simulink model "RobotX_ss_acousticsSKIP_dock_odoa_ta_1021"  (R2014a)
settings: Solver=FixedStepDiscrete  StartTime=0.0  StopTime=inf  FixedStep=.25  RelTol=1e-3
undefined symbols (not defined in the file): Com1, Com2, Com3, Com4, DiscIntNeverNeededParam, standard
libraries: xpcseriallib x42, simulink x8, slrtlib x8, speedgoatlib x2, speedgoatlib_IO102 x1
(part 6 of 19)

== matlab function RobotX_ss_acousticsSKIP_dock_odoa_ta_1021/Main FSM/ODOA/SLAM1/Models for prediction/Model36/Dynamic Model ==
  data: F_surge input; F_sway input; Torque input; u input; surgeAccel output; v input; psi input; swayAccel output; yawAccel output
function [surgeAccel, swayAccel, yawAccel] = ...
    WAM_V_3DOF(F_surge, F_sway, Torque, u, v, psi)
%Written by Anderson Lebbad on August 12, 2014
%Last Edited:

%This function was heavily based off of Ariel Qu's Vel3DOF_IvanV1. It was
%rewritten for real-time use.

%This function will produce the transient output surge velocity of a
%linearized model of the USV. It is assumed that the vehicle is equivalent
%to two cylinders in the water.

%%%%%DEFINED VARIABLE%%%%%%
%
%   Xext = Thrust from motors
%   Next = Moment from motor
%   m = Mass of vehicle
%   Xudot = Added mass in surge direction
%   Yvdot = Added mass in sway direction
%   Nrdot = Added mass from yaw
%   xg = offset from center of gravity
%   rho = density of seawater
%   S = wetted surface area
%   R = Reynolds number
%   Cd = Coefficient of drag
%   Cdc = Coefficient of drag for sway
%   nu = Kinematic viscosity
%   L = Length overall
%   T = draft
%   B = beam
%   SA = Surface area of cylinder experiencing sway
%   Iz = moment of inertia about Z axis
%
%%%%%%

% Force/Mometns from thrusters & control surfaces...

tau = [F_surge; F_sway; Torque];

% Calculate yaw rate
persistent lastHeading
if isempty(lastHeading)
    lastHeading = psi;
end
%Sample time
ts = .1;

r = (psi - lastHeading)/ts;

% Velocity & Angular velocity vectors
vel = [u; v; 0];
omega = [0; 0; r];

%define variables
m = 145.7;         % Total mass [kg] - reduced from 102
rho = 1025.9;   % density of seawater [kg/m^3]
L = 3.91*0.85;  % Length on the waterline [m]
B = 0.426;       % Demihull beam [m]
T = B*0.2;        % Draft of the demihull [m]
p_bar = 1.0; % sidehull separation - from centerplane vessel to centerplane demihull
Iz = 262.181;    % Mass moment of inertia about z-axis [kg*m^2]
xg = 0;         % Body-Fixed coordinate system taken to be center of gravity
yg = 0;         % Symmetrical Vessel
Cd = 1.1;       % Drag coefficient for a lateral cylinder
LCG = 1.485;        % Need to know where LCG wrt stern

% Vector location of port and starboard hulls
r_port = [-LCG; -p_bar; 0];   
r_stbd = [-LCG; p_bar; 0];

% Port and starboard hull velocities
vel_port = vel + cross(omega,r_port);
vel_stbd = vel + cross(omega,r_stbd);

u_port = vel_port(1);
u_stbd = vel_stbd(1);

% Port and starboard state vectors
state_port = vel_port + omega;
state_stbd = vel_stbd + omega;

%% Added Mass
% Estimated for each hull, then multiplied by 2 to account for both hulls
Xudot = -0.05*m;

%Using strip theory to estimate added mass coefficients
Nrdot = -(4.75/2*pi*rho*p_bar*T^4 + pi*rho*T^2*((L - LCG)^3 + LCG^3)/3);
Nvdot = - pi*rho*T^2*((L - LCG)^2 - LCG^2)/2;

Yrdot = Nvdot;
Yvdot = -rho*pi*T^2*L;

% Multiply by 2:
Xudot = 2*Xudot;
Nrdot = 2*Nrdot;
Nvdot = 2*Nvdot;
Yrdot = 2*Yrdot;
Yvdot = 2*Yvdot;

%Calculate Coefficient of Drag for Sway from 1950 SNAME approximation
Cdc= 1.1 + 0.0045*L/T - 0.1*B/T + 0.016*(B/T)^2;
SA = 2*pi/4*T*L; %projected area of pontoon for two pontoons

%% Linear Drag Terms
%Total Speed
U = sqrt(u^2+v^2);

Xu = 0;
Yv = -0.5*rho*abs(v)*2*Cdc*SA; %20 was the last working number %from SNAME 1950, x2 for two cylinders
%Nr = -0.5*pi*rho*U*T^2*L^2;
Nr = -pi*rho*U*T^2*L^2*.065;
Nv = -pi*rho*U*T^2*L*.01;
Yr = pi*rho*U*T^2*L*0.2;  %from Newman approximation in Lewandowski

%% Nonlinear Drag Terms

% Drag and Moment due to drag on entire vessel - includes nonlinear and
% linear drag terms
D_port = 0.5*(0.44*u_port^3 - 0.01*u_port^2 + 19*u_port);     % Can assume that this equation also takes into account Xu - so set Xu=0
D_stbd = 0.5*(0.44*u_stbd^3 - 0.01*u_stbd^2 + 19*u_stbd);     % Can assume that this equation also takes into account Xu - so set Xu=0

tau_drag = [-(D_port + D_stbd); 0; (D_stbd - D_port)*p_bar];

Xuu = 0;

%% Maneuvering Coefficient Matrices
% Added Mass Matrix
M = [(m - Xudot)      0              0;...
    0               (m - Yvdot)     (m*xg - Yrdot);...
    0               (m*xg - Nvdot)  (Iz - Nrdot)];

%Centripetal and Added Mass Centripetal force matrices
% C_RB = [
%     0                  0                0
%     0                  0                0
%     0                  0                0
%     ];

% C_RB = [
%     0                  0                -m*(xg*r + v)
%     0                  0                -m*(yg*r - u)
%     m*(xg*r + v)       m*(yg*r - u)     0
%     ];

% C_A = -[ %negative originally
%     0                               0           0
%     0                               0           0
%     0                               0           0
%     ];

% Negating centripetal acceleration for test
C_RB = 0;
C_A = 0;

D = -[Xu  0   0;...
      0   Yv  Yr;...
      0   Nv  Nr];

% Nonlinear Drag Coefficients
D_N = -[Xuu*u   0                       0;...
        0       0                       0;...
        0       0                       0];
    
%% Calculate the port and starboard force vectors
tau_port = -(C_RB + C_A + D + D_N)*state_port;
tau_stbd = -(C_RB + C_A + D + D_N)*state_stbd;


%% Sum the force vectors
tau_tot = tau + tau_drag + tau_port + tau_stbd...
    + cross(r_port,[tau_port(1);tau_port(2);0]) + ...
    cross(r_stbd,[tau_stbd(1);tau_stbd(2);0]);

% Calculate the time derivative of the state vector

accel = M\tau_tot;

%% Separate output

surgeAccel = accel(1);
swayAccel = accel(2);
yawAccel = accel(3);

end

== matlab function RobotX_ss_acousticsSKIP_dock_odoa_ta_1021/Main FSM/ODOA/SLAM1/Models for prediction/Model39/Stbd Thruster Model ==
  data: stbdMP input; F_surge output; stbdAzimuth input; F_sway output; Torque output
function [F_surge,F_sway,Torque]  = StarBoardThruster(stbdMP,stbdAzimuth)
%Approximation for Starboard Force and Moment with the input motor power
%and azimuth angle of thruster

%Longitudinal distance from center of mass
longDist =1.007;           %m

%Axial distance from center of mass
axialDist=1.485;            %m

%% Piece-wise thrust calculation

if stbdMP <= -51.0119
    F = .9140*stbdMP + 40;
elseif stbdMP >= 26.8367
    F = 1.658*stbdMP - 41.01;
else
    F = .12987*stbdMP;
end

%% Force components
F_surge=F*cos(stbdAzimuth*pi/180);       %N
F_sway=F*sin(stbdAzimuth*pi/180);       %N

%% Torque calculation

Torque = -F_surge*longDist - F_sway*axialDist;   %N.m

end

== matlab function RobotX_ss_acousticsSKIP_dock_odoa_ta_1021/Main FSM/ODOA/SLAM1/Models for prediction/Model4/Dynamic Model ==
  data: F_surge input; F_sway input; Torque input; u input; surgeAccel output; v input; psi input; swayAccel output; yawAccel output
function [surgeAccel, swayAccel, yawAccel] = ...
    WAM_V_3DOF(F_surge, F_sway, Torque, u, v, psi)
%Written by Anderson Lebbad on August 12, 2014
%Last Edited:

%This function was heavily based off of Ariel Qu's Vel3DOF_IvanV1. It was
%rewritten for real-time use.

%This function will produce the transient output surge velocity of a
%linearized model of the USV. It is assumed that the vehicle is equivalent
%to two cylinders in the water.

%%%%%DEFINED VARIABLE%%%%%%
%
%   Xext = Thrust from motors
%   Next = Moment from motor
%   m = Mass of vehicle
%   Xudot = Added mass in surge direction
%   Yvdot = Added mass in sway direction
%   Nrdot = Added mass from yaw
%   xg = offset from center of gravity
%   rho = density of seawater
%   S = wetted surface area
%   R = Reynolds number
%   Cd = Coefficient of drag
%   Cdc = Coefficient of drag for sway
%   nu = Kinematic viscosity
%   L = Length overall
%   T = draft
%   B = beam
%   SA = Surface area of cylinder experiencing sway
%   Iz = moment of inertia about Z axis
%
%%%%%%

% Force/Mometns from thrusters & control surfaces...

tau = [F_surge; F_sway; Torque];

% Calculate yaw rate
persistent lastHeading
if isempty(lastHeading)
    lastHeading = psi;
end
%Sample time
ts = .1;

r = (psi - lastHeading)/ts;

% Velocity & Angular velocity vectors
vel = [u; v; 0];
omega = [0; 0; r];

%define variables
m = 145.7;         % Total mass [kg] - reduced from 102
rho = 1025.9;   % density of seawater [kg/m^3]
L = 3.91*0.85;  % Length on the waterline [m]
B = 0.426;       % Demihull beam [m]
T = B*0.2;        % Draft of the demihull [m]
p_bar = 1.0; % sidehull separation - from centerplane vessel to centerplane demihull
Iz = 262.181;    % Mass moment of inertia about z-axis [kg*m^2]
xg = 0;         % Body-Fixed coordinate system taken to be center of gravity
yg = 0;         % Symmetrical Vessel
Cd = 1.1;       % Drag coefficient for a lateral cylinder
LCG = 1.485;        % Need to know where LCG wrt stern

% Vector location of port and starboard hulls
r_port = [-LCG; -p_bar; 0];   
r_stbd = [-LCG; p_bar; 0];

% Port and starboard hull velocities
vel_port = vel + cross(omega,r_port);
vel_stbd = vel + cross(omega,r_stbd);

u_port = vel_port(1);
u_stbd = vel_stbd(1);

% Port and starboard state vectors
state_port = vel_port + omega;
state_stbd = vel_stbd + omega;

%% Added Mass
% Estimated for each hull, then multiplied by 2 to account for both hulls
Xudot = -0.05*m;

%Using strip theory to estimate added mass coefficients
Nrdot = -(4.75/2*pi*rho*p_bar*T^4 + pi*rho*T^2*((L - LCG)^3 + LCG^3)/3);
Nvdot = - pi*rho*T^2*((L - LCG)^2 - LCG^2)/2;

Yrdot = Nvdot;
Yvdot = -rho*pi*T^2*L;

% Multiply by 2:
Xudot = 2*Xudot;
Nrdot = 2*Nrdot;
Nvdot = 2*Nvdot;
Yrdot = 2*Yrdot;
Yvdot = 2*Yvdot;

%Calculate Coefficient of Drag for Sway from 1950 SNAME approximation
Cdc= 1.1 + 0.0045*L/T - 0.1*B/T + 0.016*(B/T)^2;
SA = 2*pi/4*T*L; %projected area of pontoon for two pontoons

%% Linear Drag Terms
%Total Speed
U = sqrt(u^2+v^2);

Xu = 0;
Yv = -0.5*rho*abs(v)*2*Cdc*SA; %20 was the last working number %from SNAME 1950, x2 for two cylinders
%Nr = -0.5*pi*rho*U*T^2*L^2;
Nr = -pi*rho*U*T^2*L^2*.065;
Nv = -pi*rho*U*T^2*L*.01;
Yr = pi*rho*U*T^2*L*0.2;  %from Newman approximation in Lewandowski

%% Nonlinear Drag Terms

% Drag and Moment due to drag on entire vessel - includes nonlinear and
% linear drag terms
D_port = 0.5*(0.44*u_port^3 - 0.01*u_port^2 + 19*u_port);     % Can assume that this equation also takes into account Xu - so set Xu=0
D_stbd = 0.5*(0.44*u_stbd^3 - 0.01*u_stbd^2 + 19*u_stbd);     % Can assume that this equation also takes into account Xu - so set Xu=0

tau_drag = [-(D_port + D_stbd); 0; (D_stbd - D_port)*p_bar];

Xuu = 0;

%% Maneuvering Coefficient Matrices
% Added Mass Matrix
M = [(m - Xudot)      0              0;...
    0               (m - Yvdot)     (m*xg - Yrdot);...
    0               (m*xg - Nvdot)  (Iz - Nrdot)];

%Centripetal and Added Mass Centripetal force matrices
% C_RB = [
%     0                  0                0
%     0                  0                0
%     0                  0                0
%     ];

% C_RB = [
%     0                  0                -m*(xg*r + v)
%     0                  0                -m*(yg*r - u)
%     m*(xg*r + v)       m*(yg*r - u)     0
%     ];

% C_A = -[ %negative originally
%     0                               0           0
%     0                               0           0
%     0                               0           0
%     ];

% Negating centripetal acceleration for test
C_RB = 0;
C_A = 0;

D = -[Xu  0   0;...
      0   Yv  Yr;...
      0   Nv  Nr];

% Nonlinear Drag Coefficients
D_N = -[Xuu*u   0                       0;...
        0       0                       0;...
        0       0                       0];
    
%% Calculate the port and starboard force vectors
tau_port = -(C_RB + C_A + D + D_N)*state_port;
tau_stbd = -(C_RB + C_A + D + D_N)*state_stbd;


%% Sum the force vectors
tau_tot = tau + tau_drag + tau_port + tau_stbd...
    + cross(r_port,[tau_port(1);tau_port(2);0]) + ...
    cross(r_stbd,[tau_stbd(1);tau_stbd(2);0]);

% Calculate the time derivative of the state vector

accel = M\tau_tot;

%% Separate output

surgeAccel = accel(1);
swayAccel = accel(2);
yawAccel = accel(3);

end

== matlab function RobotX_ss_acousticsSKIP_dock_odoa_ta_1021/Main FSM/ODOA/SLAM1/Models for prediction/Model42/Stbd Thruster Model ==
  data: stbdMP input; F_surge output; stbdAzimuth input; F_sway output; Torque output
function [F_surge,F_sway,Torque]  = StarBoardThruster(stbdMP,stbdAzimuth)
%Approximation for Starboard Force and Moment with the input motor power
%and azimuth angle of thruster

%Longitudinal distance from center of mass
longDist =1.007;           %m

%Axial distance from center of mass
axialDist=1.485;            %m

%% Piece-wise thrust calculation

if stbdMP <= -51.0119
    F = .9140*stbdMP + 40;
elseif stbdMP >= 26.8367
    F = 1.658*stbdMP - 41.01;
else
    F = .12987*stbdMP;
end

%% Force components
F_surge=F*cos(stbdAzimuth*pi/180);       %N
F_sway=F*sin(stbdAzimuth*pi/180);       %N

%% Torque calculation

Torque = -F_surge*longDist - F_sway*axialDist;   %N.m

end

== matlab function RobotX_ss_acousticsSKIP_dock_odoa_ta_1021/Main FSM/ODOA/SLAM1/Models for prediction/Model43/Non-Holonomic Constraint ==
  data: time input; surgeAccel input; NEyaw output; swayAccel input; YawAccel input; u input; v input; gyrz input; psi input; X input; Y input
function NEyaw  = nonHolonomicNE(time,surgeAccel,swayAccel,YawAccel,u,v,gyrz,psi,X,Y)
%Written by Anderson Lebbad on August 12, 2014
%Last Edited:

%This function estimates the velocities for a new pose based off the 
%velocities and heading calculated from the dynamic model, and the current 
%pose. Uses a non-holonomic constraint for estimation.

%% Find time elapsed for integration

ts = .1;
persistent uPrev vPrev gyrzPrev psiPrev xPrev yPrev

%Initialize
if isempty(uPrev)
    uPrev = [u time];
    vPrev = [v time];
    gyrzPrev = [gyrz time];
    psiPrev = [psi time];
    xPrev = [X time];
    yPrev = [Y time];
end
    
%Update if change
if uPrev(1) ~= u
    uPrev = [u time];
end
if vPrev(1) ~= v
    vPrev = [v time];
end
if gyrzPrev(1) ~= gyrz
    gyrzPrev = [gyrz time];
end
if psiPrev(1) ~= psi
    psiPrev = [psi time];
end
if xPrev(1) ~= X
    xPrev = [X time];
end
if yPrev(1) ~= Y
    yPrev = [Y time];
end

%evaluate elapsed
uTime = ts + time - uPrev(2);
vTime = ts + time - vPrev(2);
gyrzTime = ts + time - gyrzPrev(2);
psiTime = ts + time - psiPrev(2);
xTime = ts + time - xPrev(2);
yTime = ts + time - yPrev(2);

%% Integrate inputs
surgeVel = u + surgeAccel*uTime/2;
swayVel = v + swayAccel*vTime/2;
yawVel = gyrz + YawAccel*gyrzTime/2;
yaw = psi + yawVel*psiTime/2;


%% Apply Non-holonomic constraint for NE velocities
Xd = surgeVel*cos(yaw*pi/180) - swayVel*sin(yaw*pi/180);
Yd = surgeVel*sin(yaw*pi/180) + swayVel*cos(yaw*pi/180);

%% Integrate to output NE coordinates
N = X + Xd*xTime/2;
E = Y + Yd*yTime/2;

NEyaw = [N;E;yaw];

end

== matlab function RobotX_ss_acousticsSKIP_dock_odoa_ta_1021/Main FSM/ODOA/SLAM1/Models for prediction/Model44/Port Thruster Model ==
  data: portMP input; F_surge output; portAzimuth input; F_sway output; Torque output
function [F_surge,F_sway,Torque]  = PortThruster(portMP,portAzimuth)
%Approximation for Starboard Force and Moment with the input motor power
%and azimuth angle of thruster

%Longitudinal distance from center of mass
longDist =1.007;           %m

%Axial distance from center of mass
axialDist=1.485;            %m

%% Piece-wise thrust calculation

if portMP <= -51.0119
    F = .9140*portMP + 40;
elseif portMP >= 26.8367
    F = 1.658*portMP - 41.01;
else
    F = .12987*portMP;
end

%% Force components
F_surge=F*cos(portAzimuth*pi/180);       %N
F_sway=F*sin(portAzimuth*pi/180);       %N

%% Torque calculation

Torque = F_surge*longDist - F_sway*axialDist;   %N.m

end

== matlab function RobotX_ss_acousticsSKIP_dock_odoa_ta_1021/Main FSM/ODOA/SLAM1/Models for prediction/Model44/move_part ==
  data: PtThrust input; portMP output; PtAzimuth input; StThrust input; StAzimuth input; noiseLevel input; portAzimuth output; stbdMP output; stbdAzimuth output
function [portMP,portAzimuth,stbdMP,stbdAzimuth] = addNoise(PtThrust,...
    PtAzimuth,StThrust,StAzimuth,noiseLevel)
%Written By Anderson Lebbad on September 16, 2014
%Last Edited By:

%This function adds gaussian noise to the inputs for a particular particles
%model

portMP = normrnd(PtThrust, noiseLevel);
portAzimuth = normrnd(PtAzimuth, noiseLevel);
stbdMP = normrnd(StThrust, noiseLevel);
stbdAzimuth = normrnd(StAzimuth, noiseLevel);

end

== matlab function RobotX_ss_acousticsSKIP_dock_odoa_ta_1021/Main FSM/ODOA/SLAM1/Models for prediction/Model45/Dynamic Model ==
  data: F_surge input; F_sway input; Torque input; u input; surgeAccel output; v input; psi input; swayAccel output; yawAccel output
function [surgeAccel, swayAccel, yawAccel] = ...
    WAM_V_3DOF(F_surge, F_sway, Torque, u, v, psi)
%Written by Anderson Lebbad on August 12, 2014
%Last Edited:

%This function was heavily based off of Ariel Qu's Vel3DOF_IvanV1. It was
%rewritten for real-time use.

%This function will produce the transient output surge velocity of a
%linearized model of the USV. It is assumed that the vehicle is equivalent
%to two cylinders in the water.

%%%%%DEFINED VARIABLE%%%%%%
%
%   Xext = Thrust from motors
%   Next = Moment from motor
%   m = Mass of vehicle
%   Xudot = Added mass in surge direction
%   Yvdot = Added mass in sway direction
%   Nrdot = Added mass from yaw
%   xg = offset from center of gravity
%   rho = density of seawater
%   S = wetted surface area
%   R = Reynolds number
%   Cd = Coefficient of drag
%   Cdc = Coefficient of drag for sway
%   nu = Kinematic viscosity
%   L = Length overall
%   T = draft
%   B = beam
%   SA = Surface area of cylinder experiencing sway
%   Iz = moment of inertia about Z axis
%
%%%%%%

% Force/Mometns from thrusters & control surfaces...

tau = [F_surge; F_sway; Torque];

% Calculate yaw rate
persistent lastHeading
if isempty(lastHeading)
    lastHeading = psi;
end
%Sample time
ts = .1;

r = (psi - lastHeading)/ts;

% Velocity & Angular velocity vectors
vel = [u; v; 0];
omega = [0; 0; r];

%define variables
m = 145.7;         % Total mass [kg] - reduced from 102
rho = 1025.9;   % density of seawater [kg/m^3]
L = 3.91*0.85;  % Length on the waterline [m]
B = 0.426;       % Demihull beam [m]
T = B*0.2;        % Draft of the demihull [m]
p_bar = 1.0; % sidehull separation - from centerplane vessel to centerplane demihull
Iz = 262.181;    % Mass moment of inertia about z-axis [kg*m^2]
xg = 0;         % Body-Fixed coordinate system taken to be center of gravity
yg = 0;         % Symmetrical Vessel
Cd = 1.1;       % Drag coefficient for a lateral cylinder
LCG = 1.485;        % Need to know where LCG wrt stern

% Vector location of port and starboard hulls
r_port = [-LCG; -p_bar; 0];   
r_stbd = [-LCG; p_bar; 0];

% Port and starboard hull velocities
vel_port = vel + cross(omega,r_port);
vel_stbd = vel + cross(omega,r_stbd);

u_port = vel_port(1);
u_stbd = vel_stbd(1);

% Port and starboard state vectors
state_port = vel_port + omega;
state_stbd = vel_stbd + omega;

%% Added Mass
% Estimated for each hull, then multiplied by 2 to account for both hulls
Xudot = -0.05*m;

%Using strip theory to estimate added mass coefficients
Nrdot = -(4.75/2*pi*rho*p_bar*T^4 + pi*rho*T^2*((L - LCG)^3 + LCG^3)/3);
Nvdot = - pi*rho*T^2*((L - LCG)^2 - LCG^2)/2;

Yrdot = Nvdot;
Yvdot = -rho*pi*T^2*L;

% Multiply by 2:
Xudot = 2*Xudot;
Nrdot = 2*Nrdot;
Nvdot = 2*Nvdot;
Yrdot = 2*Yrdot;
Yvdot = 2*Yvdot;

%Calculate Coefficient of Drag for Sway from 1950 SNAME approximation
Cdc= 1.1 + 0.0045*L/T - 0.1*B/T + 0.016*(B/T)^2;
SA = 2*pi/4*T*L; %projected area of pontoon for two pontoons

%% Linear Drag Terms
%Total Speed
U = sqrt(u^2+v^2);

Xu = 0;
Yv = -0.5*rho*abs(v)*2*Cdc*SA; %20 was the last working number %from SNAME 1950, x2 for two cylinders
%Nr = -0.5*pi*rho*U*T^2*L^2;
Nr = -pi*rho*U*T^2*L^2*.065;
Nv = -pi*rho*U*T^2*L*.01;
Yr = pi*rho*U*T^2*L*0.2;  %from Newman approximation in Lewandowski

%% Nonlinear Drag Terms

% Drag and Moment due to drag on entire vessel - includes nonlinear and
% linear drag terms
D_port = 0.5*(0.44*u_port^3 - 0.01*u_port^2 + 19*u_port);     % Can assume that this equation also takes into account Xu - so set Xu=0
D_stbd = 0.5*(0.44*u_stbd^3 - 0.01*u_stbd^2 + 19*u_stbd);     % Can assume that this equation also takes into account Xu - so set Xu=0

tau_drag = [-(D_port + D_stbd); 0; (D_stbd - D_port)*p_bar];

Xuu = 0;

%% Maneuvering Coefficient Matrices
% Added Mass Matrix
M = [(m - Xudot)      0              0;...
    0               (m - Yvdot)     (m*xg - Yrdot);...
    0               (m*xg - Nvdot)  (Iz - Nrdot)];

%Centripetal and Added Mass Centripetal force matrices
% C_RB = [
%     0                  0                0
%     0                  0                0
%     0                  0                0
%     ];

% C_RB = [
%     0                  0                -m*(xg*r + v)
%     0                  0                -m*(yg*r - u)
%     m*(xg*r + v)       m*(yg*r - u)     0
%     ];

% C_A = -[ %negative originally
%     0                               0           0
%     0                               0           0
%     0                               0           0
%     ];

% Negating centripetal acceleration for test
C_RB = 0;
C_A = 0;

D = -[Xu  0   0;...
      0   Yv  Yr;...
      0   Nv  Nr];

% Nonlinear Drag Coefficients
D_N = -[Xuu*u   0                       0;...
        0       0                       0;...
        0       0                       0];
    
%% Calculate the port and starboard force vectors
tau_port = -(C_RB + C_A + D + D_N)*state_port;
tau_stbd = -(C_RB + C_A + D + D_N)*state_stbd;


%% Sum the force vectors
tau_tot = tau + tau_drag + tau_port + tau_stbd...
    + cross(r_port,[tau_port(1);tau_port(2);0]) + ...
    cross(r_stbd,[tau_stbd(1);tau_stbd(2);0]);

% Calculate the time derivative of the state vector

accel = M\tau_tot;

%% Separate output

surgeAccel = accel(1);
swayAccel = accel(2);
yawAccel = accel(3);

end

== matlab function RobotX_ss_acousticsSKIP_dock_odoa_ta_1021/Main FSM/ODOA/SLAM1/Models for prediction/Model48/Stbd Thruster Model ==
  data: stbdMP input; F_surge output; stbdAzimuth input; F_sway output; Torque output
function [F_surge,F_sway,Torque]  = StarBoardThruster(stbdMP,stbdAzimuth)
%Approximation for Starboard Force and Moment with the input motor power
%and azimuth angle of thruster

%Longitudinal distance from center of mass
longDist =1.007;           %m

%Axial distance from center of mass
axialDist=1.485;            %m

%% Piece-wise thrust calculation

if stbdMP <= -51.0119
    F = .9140*stbdMP + 40;
elseif stbdMP >= 26.8367
    F = 1.658*stbdMP - 41.01;
else
    F = .12987*stbdMP;
end

%% Force components
F_surge=F*cos(stbdAzimuth*pi/180);       %N
F_sway=F*sin(stbdAzimuth*pi/180);       %N

%% Torque calculation

Torque = -F_surge*longDist - F_sway*axialDist;   %N.m

end

== matlab function RobotX_ss_acousticsSKIP_dock_odoa_ta_1021/Main FSM/ODOA/SLAM1/Models for prediction/Model49/Dynamic Model ==
  data: F_surge input; F_sway input; Torque input; u input; surgeAccel output; v input; psi input; swayAccel output; yawAccel output
function [surgeAccel, swayAccel, yawAccel] = ...
    WAM_V_3DOF(F_surge, F_sway, Torque, u, v, psi)
%Written by Anderson Lebbad on August 12, 2014
%Last Edited:

%This function was heavily based off of Ariel Qu's Vel3DOF_IvanV1. It was
%rewritten for real-time use.

%This function will produce the transient output surge velocity of a
%linearized model of the USV. It is assumed that the vehicle is equivalent
%to two cylinders in the water.

%%%%%DEFINED VARIABLE%%%%%%
%
%   Xext = Thrust from motors
%   Next = Moment from motor
%   m = Mass of vehicle
%   Xudot = Added mass in surge direction
%   Yvdot = Added mass in sway direction
%   Nrdot = Added mass from yaw
%   xg = offset from center of gravity
%   rho = density of seawater
%   S = wetted surface area
%   R = Reynolds number
%   Cd = Coefficient of drag
%   Cdc = Coefficient of drag for sway
%   nu = Kinematic viscosity
%   L = Length overall
%   T = draft
%   B = beam
%   SA = Surface area of cylinder experiencing sway
%   Iz = moment of inertia about Z axis
%
%%%%%%

% Force/Mometns from thrusters & control surfaces...

tau = [F_surge; F_sway; Torque];

% Calculate yaw rate
persistent lastHeading
if isempty(lastHeading)
    lastHeading = psi;
end
%Sample time
ts = .1;

r = (psi - lastHeading)/ts;

% Velocity & Angular velocity vectors
vel = [u; v; 0];
omega = [0; 0; r];

%define variables
m = 145.7;         % Total mass [kg] - reduced from 102
rho = 1025.9;   % density of seawater [kg/m^3]
L = 3.91*0.85;  % Length on the waterline [m]
B = 0.426;       % Demihull beam [m]
T = B*0.2;        % Draft of the demihull [m]
p_bar = 1.0; % sidehull separation - from centerplane vessel to centerplane demihull
Iz = 262.181;    % Mass moment of inertia about z-axis [kg*m^2]
xg = 0;         % Body-Fixed coordinate system taken to be center of gravity
yg = 0;         % Symmetrical Vessel
Cd = 1.1;       % Drag coefficient for a lateral cylinder
LCG = 1.485;        % Need to know where LCG wrt stern

% Vector location of port and starboard hulls
r_port = [-LCG; -p_bar; 0];   
r_stbd = [-LCG; p_bar; 0];

% Port and starboard hull velocities
vel_port = vel + cross(omega,r_port);
vel_stbd = vel + cross(omega,r_stbd);

u_port = vel_port(1);
u_stbd = vel_stbd(1);

% Port and starboard state vectors
state_port = vel_port + omega;
state_stbd = vel_stbd + omega;

%% Added Mass
% Estimated for each hull, then multiplied by 2 to account for both hulls
Xudot = -0.05*m;

%Using strip theory to estimate added mass coefficients
Nrdot = -(4.75/2*pi*rho*p_bar*T^4 + pi*rho*T^2*((L - LCG)^3 + LCG^3)/3);
Nvdot = - pi*rho*T^2*((L - LCG)^2 - LCG^2)/2;

Yrdot = Nvdot;
Yvdot = -rho*pi*T^2*L;

% Multiply by 2:
Xudot = 2*Xudot;
Nrdot = 2*Nrdot;
Nvdot = 2*Nvdot;
Yrdot = 2*Yrdot;
Yvdot = 2*Yvdot;

%Calculate Coefficient of Drag for Sway from 1950 SNAME approximation
Cdc= 1.1 + 0.0045*L/T - 0.1*B/T + 0.016*(B/T)^2;
SA = 2*pi/4*T*L; %projected area of pontoon for two pontoons

%% Linear Drag Terms
%Total Speed
U = sqrt(u^2+v^2);

Xu = 0;
Yv = -0.5*rho*abs(v)*2*Cdc*SA; %20 was the last working number %from SNAME 1950, x2 for two cylinders
%Nr = -0.5*pi*rho*U*T^2*L^2;
Nr = -pi*rho*U*T^2*L^2*.065;
Nv = -pi*rho*U*T^2*L*.01;
Yr = pi*rho*U*T^2*L*0.2;  %from Newman approximation in Lewandowski

%% Nonlinear Drag Terms

% Drag and Moment due to drag on entire vessel - includes nonlinear and
% linear drag terms
D_port = 0.5*(0.44*u_port^3 - 0.01*u_port^2 + 19*u_port);     % Can assume that this equation also takes into account Xu - so set Xu=0
D_stbd = 0.5*(0.44*u_stbd^3 - 0.01*u_stbd^2 + 19*u_stbd);     % Can assume that this equation also takes into account Xu - so set Xu=0

tau_drag = [-(D_port + D_stbd); 0; (D_stbd - D_port)*p_bar];

Xuu = 0;

%% Maneuvering Coefficient Matrices
% Added Mass Matrix
M = [(m - Xudot)      0              0;...
    0               (m - Yvdot)     (m*xg - Yrdot);...
    0               (m*xg - Nvdot)  (Iz - Nrdot)];

%Centripetal and Added Mass Centripetal force matrices
% C_RB = [
%     0                  0                0
%     0                  0                0
%     0                  0                0
%     ];

% C_RB = [
%     0                  0                -m*(xg*r + v)
%     0                  0                -m*(yg*r - u)
%     m*(xg*r + v)       m*(yg*r - u)     0
%     ];

% C_A = -[ %negative originally
%     0                               0           0
%     0                               0           0
%     0                               0           0
%     ];

% Negating centripetal acceleration for test
C_RB = 0;
C_A = 0;

D = -[Xu  0   0;...
      0   Yv  Yr;...
      0   Nv  Nr];

% Nonlinear Drag Coefficients
D_N = -[Xuu*u   0                       0;...
        0       0                       0;...
        0       0                       0];
    
%% Calculate the port and starboard force vectors
tau_port = -(C_RB + C_A + D + D_N)*state_port;
tau_stbd = -(C_RB + C_A + D + D_N)*state_stbd;


%% Sum the force vectors
tau_tot = tau + tau_drag + tau_port + tau_stbd...
    + cross(r_port,[tau_port(1);tau_port(2);0]) + ...
    cross(r_stbd,[tau_stbd(1);tau_stbd(2);0]);

% Calculate the time derivative of the state vector

accel = M\tau_tot;

%% Separate output

surgeAccel = accel(1);
swayAccel = accel(2);
yawAccel = accel(3);

end

== matlab function RobotX_ss_acousticsSKIP_dock_odoa_ta_1021/Main FSM/ODOA/SLAM1/Models for prediction/Model6/Stbd Thruster Model ==
  data: stbdMP input; F_surge output; stbdAzimuth input; F_sway output; Torque output
function [F_surge,F_sway,Torque]  = StarBoardThruster(stbdMP,stbdAzimuth)
%Approximation for Starboard Force and Moment with the input motor power
%and azimuth angle of thruster

%Longitudinal distance from center of mass
longDist =1.007;           %m

%Axial distance from center of mass
axialDist=1.485;            %m

%% Piece-wise thrust calculation

if stbdMP <= -51.0119
    F = .9140*stbdMP + 40;
elseif stbdMP >= 26.8367
    F = 1.658*stbdMP - 41.01;
else
    F = .12987*stbdMP;
end

%% Force components
F_surge=F*cos(stbdAzimuth*pi/180);       %N
F_sway=F*sin(stbdAzimuth*pi/180);       %N

%% Torque calculation

Torque = -F_surge*longDist - F_sway*axialDist;   %N.m

end

== matlab function RobotX_ss_acousticsSKIP_dock_odoa_ta_1021/Main FSM/ODOA/SLAM1/Models for prediction/Model7/Dynamic Model ==
  data: F_surge input; F_sway input; Torque input; u input; surgeAccel output; v input; psi input; swayAccel output; yawAccel output
function [surgeAccel, swayAccel, yawAccel] = ...
    WAM_V_3DOF(F_surge, F_sway, Torque, u, v, psi)
%Written by Anderson Lebbad on August 12, 2014
%Last Edited:

%This function was heavily based off of Ariel Qu's Vel3DOF_IvanV1. It was
%rewritten for real-time use.

%This function will produce the transient output surge velocity of a
%linearized model of the USV. It is assumed that the vehicle is equivalent
%to two cylinders in the water.

%%%%%DEFINED VARIABLE%%%%%%
%
%   Xext = Thrust from motors
%   Next = Moment from motor
%   m = Mass of vehicle
%   Xudot = Added mass in surge direction
%   Yvdot = Added mass in sway direction
%   Nrdot = Added mass from yaw
%   xg = offset from center of gravity
%   rho = density of seawater
%   S = wetted surface area
%   R = Reynolds number
%   Cd = Coefficient of drag
%   Cdc = Coefficient of drag for sway
%   nu = Kinematic viscosity
%   L = Length overall
%   T = draft
%   B = beam
%   SA = Surface area of cylinder experiencing sway
%   Iz = moment of inertia about Z axis
%
%%%%%%

% Force/Mometns from thrusters & control surfaces...

tau = [F_surge; F_sway; Torque];

% Calculate yaw rate
persistent lastHeading
if isempty(lastHeading)
    lastHeading = psi;
end
%Sample time
ts = .1;

r = (psi - lastHeading)/ts;

% Velocity & Angular velocity vectors
vel = [u; v; 0];
omega = [0; 0; r];

%define variables
m = 145.7;         % Total mass [kg] - reduced from 102
rho = 1025.9;   % density of seawater [kg/m^3]
L = 3.91*0.85;  % Length on the waterline [m]
B = 0.426;       % Demihull beam [m]
T = B*0.2;        % Draft of the demihull [m]
p_bar = 1.0; % sidehull separation - from centerplane vessel to centerplane demihull
Iz = 262.181;    % Mass moment of inertia about z-axis [kg*m^2]
xg = 0;         % Body-Fixed coordinate system taken to be center of gravity
yg = 0;         % Symmetrical Vessel
Cd = 1.1;       % Drag coefficient for a lateral cylinder
LCG = 1.485;        % Need to know where LCG wrt stern

% Vector location of port and starboard hulls
r_port = [-LCG; -p_bar; 0];   
r_stbd = [-LCG; p_bar; 0];

% Port and starboard hull velocities
vel_port = vel + cross(omega,r_port);
vel_stbd = vel + cross(omega,r_stbd);

u_port = vel_port(1);
u_stbd = vel_stbd(1);

% Port and starboard state vectors
state_port = vel_port + omega;
state_stbd = vel_stbd + omega;

%% Added Mass
% Estimated for each hull, then multiplied by 2 to account for both hulls
Xudot = -0.05*m;

%Using strip theory to estimate added mass coefficients
Nrdot = -(4.75/2*pi*rho*p_bar*T^4 + pi*rho*T^2*((L - LCG)^3 + LCG^3)/3);
Nvdot = - pi*rho*T^2*((L - LCG)^2 - LCG^2)/2;

Yrdot = Nvdot;
Yvdot = -rho*pi*T^2*L;

% Multiply by 2:
Xudot = 2*Xudot;
Nrdot = 2*Nrdot;
Nvdot = 2*Nvdot;
Yrdot = 2*Yrdot;
Yvdot = 2*Yvdot;

%Calculate Coefficient of Drag for Sway from 1950 SNAME approximation
Cdc= 1.1 + 0.0045*L/T - 0.1*B/T + 0.016*(B/T)^2;
SA = 2*pi/4*T*L; %projected area of pontoon for two pontoons

%% Linear Drag Terms
%Total Speed
U = sqrt(u^2+v^2);

Xu = 0;
Yv = -0.5*rho*abs(v)*2*Cdc*SA; %20 was the last working number %from SNAME 1950, x2 for two cylinders
%Nr = -0.5*pi*rho*U*T^2*L^2;
Nr = -pi*rho*U*T^2*L^2*.065;
Nv = -pi*rho*U*T^2*L*.01;
Yr = pi*rho*U*T^2*L*0.2;  %from Newman approximation in Lewandowski

%% Nonlinear Drag Terms

% Drag and Moment due to drag on entire vessel - includes nonlinear and
% linear drag terms
D_port = 0.5*(0.44*u_port^3 - 0.01*u_port^2 + 19*u_port);     % Can assume that this equation also takes into account Xu - so set Xu=0
D_stbd = 0.5*(0.44*u_stbd^3 - 0.01*u_stbd^2 + 19*u_stbd);     % Can assume that this equation also takes into account Xu - so set Xu=0

tau_drag = [-(D_port + D_stbd); 0; (D_stbd - D_port)*p_bar];

Xuu = 0;

%% Maneuvering Coefficient Matrices
% Added Mass Matrix
M = [(m - Xudot)      0              0;...
    0               (m - Yvdot)     (m*xg - Yrdot);...
    0               (m*xg - Nvdot)  (Iz - Nrdot)];

%Centripetal and Added Mass Centripetal force matrices
% C_RB = [
%     0                  0                0
%     0                  0                0
%     0                  0                0
%     ];

% C_RB = [
%     0                  0                -m*(xg*r + v)
%     0                  0                -m*(yg*r - u)
%     m*(xg*r + v)       m*(yg*r - u)     0
%     ];

% C_A = -[ %negative originally
%     0                               0           0
%     0                               0           0
%     0                               0           0
%     ];

% Negating centripetal acceleration for test
C_RB = 0;
C_A = 0;

D = -[Xu  0   0;...
      0   Yv  Yr;...
      0   Nv  Nr];

% Nonlinear Drag Coefficients
D_N = -[Xuu*u   0                       0;...
        0       0                       0;...
        0       0                       0];
    
%% Calculate the port and starboard force vectors
tau_port = -(C_RB + C_A + D + D_N)*state_port;
tau_stbd = -(C_RB + C_A + D + D_N)*state_stbd;


%% Sum the force vectors
tau_tot = tau + tau_drag + tau_port + tau_stbd...
    + cross(r_port,[tau_port(1);tau_port(2);0]) + ...
    cross(r_stbd,[tau_stbd(1);tau_stbd(2);0]);

% Calculate the time derivative of the state vector

accel = M\tau_tot;

%% Separate output

surgeAccel = accel(1);
swayAccel = accel(2);
yawAccel = accel(3);

end

== matlab function RobotX_ss_acousticsSKIP_dock_odoa_ta_1021/Main FSM/ODOA/Path/LLA to NED ==
  data: LLAs input; NEDout output; NED_origin input
function NEDout = LLA2NEDfun(LLAs,NED_origin)
%Written by Anderson Lebbad on September 20, 2014
%Last edited by:
%
%This function converts a target Latitude, Longitude, Altitude (LLA) point
%into North, East, Down (NED) coordinates

NED  = zeros(4,2);
for i=1:4
%First convert to earth centered, earth fixed frame
GoalECEF = lla2ecef([LLAs(i,:)*(pi/180), 0]');
%Then convert from ECEF to North East Down
GoalNEDvect = ecef2ned(NED_origin'*(pi/180),GoalECEF);
NED(i,:) = GoalNEDvect(1:2)';
end


%Order outputs for grid
Xord = sortrows(NED,1);
Yord = sortrows(NED,2);

BLfirst = ismember(Yord(3:4,:),Xord(3,:),'rows');
if sum(BLfirst) >= 1
    BL = Xord(3,:);
    BR = Xord(4,:);
else
    BL = Xord(4,:);
    BR = Xord(3,:);
end

TRthird = ismember(Yord(1:2,:),Xord(1,:),'rows');
if sum(TRthird) >= 1
    TR = Xord(1,:);
    TL = Xord(2,:);
else
    TR = Xord(2,:);
    TL = Xord(1,:);
end

NEDout = [BL; BR; TL; TR];

end

function x_ecef = lla2ecef(x_lla)
% LLE2ECEF: Converts from geodetic latitude, longitude, and altitude to earth-centered earth-fixed Cartesian coordinates
% INPUT: latitude phi (rad), longitude lambda (rad), altitude h (m)
% OUTPUT: [x, y, z]' (m) earth-centered earth-fixed Cartesian coordinates
    a = 6378137; % equatorial radius of ellipsoid (semi-major axis) (m)
    b = 6356752; % polar axis radius of ellipsoid (semi-minor axis) (m)

    phi = x_lla(1);
    lambda = x_lla(2);
    h = x_lla(3);
    
    % auxiliar quantities f, e, and N
    f = (a-b)/a;
    e = f*(2-f);
    N = a/sqrt(1-(e*sin(phi))^2);
    x_ecef = [(N+h)*cos(phi)*cos(lambda); (N+h)*cos(phi)*sin(lambda); (N*(1-e^2)+h)*sin(phi)];
end

function [x_ned] = ecef2ned(ned_lla, x_ecef)
% ECEF2NED Converts from earth-centered, earth-fixed Cartesian coordinates to tangent plane
% INPUT:
% 1) x_ecef=[x,y,z]' (m) earth-centered, earth-fixed Cartesian coordinates
% 2) ned_lla=[phi,lambda]' consiting of latitude phi (rad), longitude lambda (rad) of NED origin
% OUTPUT:
% 1) x_ned=[x,y,z]' (m) in NED coordinate system with the origin [phi,lambda]'

    phi = ned_lla(1);
    lambda = ned_lla(2);

    % transformation  matrix
    T = [-sin(phi)*cos(lambda) -sin(phi)*sin(lambda)  cos(phi)
         -sin(lambda)           cos(lambda)           0
          cos(phi)*cos(lambda)   cos(phi)*sin(lambda)  sin(phi)];

     x_ned = T*(x_ecef-lla2ecef([phi, lambda, 0]')); % convert to NED
     x_ned(3) = -x_ned(3);
end

== matlab function RobotX_ss_acousticsSKIP_dock_odoa_ta_1021/Main FSM/ODOA/SLAM1/Models for prediction/Model1/Port Thruster Model ==
  data: portMP input; F_surge output; portAzimuth input; F_sway output; Torque output
function [F_surge,F_sway,Torque]  = PortThruster(portMP,portAzimuth)
%Approximation for Starboard Force and Moment with the input motor power
%and azimuth angle of thruster

%Longitudinal distance from center of mass
longDist =1.007;           %m

%Axial distance from center of mass
axialDist=1.485;            %m

%% Piece-wise thrust calculation

if portMP <= -51.0119
    F = .9140*portMP + 40;
elseif portMP >= 26.8367
    F = 1.658*portMP - 41.01;
else
    F = .12987*portMP;
end

%% Force components
F_surge=F*cos(portAzimuth*pi/180);       %N
F_sway=F*sin(portAzimuth*pi/180);       %N

%% Torque calculation

Torque = F_surge*longDist - F_sway*axialDist;   %N.m

end

== system RobotX_ss_acousticsSKIP_dock_odoa_ta_1021/Main FSM/Docking/Reverse/Output Heirarchy ==
  Sensors : Inport
  Acoustic Active : Constant  Value=0
  Bus Creator2 : BusCreator  Inputs=3
  Bus Creator3 : BusCreator  Inputs=3
  Bus Creator5 : BusCreator  Inputs=2
  Constant2 : Constant  Value=[-100; -100; zeros(22,1)]
  Constant3 : Constant
  Constant4 : Constant
  Lidar Mode : Constant  Value=2
  Outputs : Outport
  wires:
  Sensors/1 -> Bus Creator5/2  "Sensors"
  Bus Creator5/1 -> Outputs/1  "Output Signals"
  Constant3/1 -> Bus Creator2/1  "Valid"
  Constant4/1 -> Bus Creator2/2  "Control Mode"
  Constant2/1 -> Bus Creator2/3  "Data"
  Bus Creator2/1 -> Bus Creator3/1  "Navigation Outputs"
  Acoustic Active/1 -> Bus Creator3/2  "Acoustic Active"
  Lidar Mode/1 -> Bus Creator3/3  "Lidar Mode"
  Bus Creator3/1 -> Bus Creator5/1  "Outputs"

== system RobotX_ss_acousticsSKIP_dock_odoa_ta_1021/Main FSM/ODOA/GPS Move/Output Reassign ==
  Vaild : Inport
  Data : Inport  Port=2
  Sensors : Inport  Port=3
  Acoustic Active : Constant  Value=0
  Bus Creator2 : BusCreator  Inputs=3
  Bus Creator3 : BusCreator  Inputs=3
  Bus Creator5 : BusCreator  Inputs=2
  Constant3 : Constant  Value=0
  Lidar Mode : Constant  Value=0
  Outputs : Outport
  wires:
  Sensors/1 -> Bus Creator5/2  "Sensors"
  Bus Creator5/1 -> Outputs/1  "Output Signals"
  Vaild/1 -> Bus Creator2/1  "Valid"
  Constant3/1 -> Bus Creator2/2  "Control Mode"
  Data/1 -> Bus Creator2/3  "Data"
  Bus Creator2/1 -> Bus Creator3/1  "Navigation Outputs"
  Acoustic Active/1 -> Bus Creator3/2  "Acoustic Active"
  Lidar Mode/1 -> Bus Creator3/3  "Lidar Mode"
  Bus Creator3/1 -> Bus Creator5/1  "Outputs"

== system RobotX_ss_acousticsSKIP_dock_odoa_ta_1021/Main FSM/ODOA/Path/Output Reassign ==
  Vaild : Inport
  Data : Inport  Port=2
  Sensors : Inport  Port=3
  Acoustic Active : Constant  Value=0
  Bus Creator2 : BusCreator  Inputs=3
  Bus Creator3 : BusCreator  Inputs=3
  Bus Creator5 : BusCreator  Inputs=2
  Constant3 : Constant  Value=0
  Lidar Mode : Constant  Value=0
  Outputs : Outport
  wires:
  Sensors/1 -> Bus Creator5/2  "Sensors"
  Bus Creator5/1 -> Outputs/1  "Output Signals"
  Vaild/1 -> Bus Creator2/1  "Valid"
  Constant3/1 -> Bus Creator2/2  "Control Mode"
  Data/1 -> Bus Creator2/3  "Data"
  Bus Creator2/1 -> Bus Creator3/1  "Navigation Outputs"
  Acoustic Active/1 -> Bus Creator3/2  "Acoustic Active"
  Lidar Mode/1 -> Bus Creator3/3  "Lidar Mode"
  Bus Creator3/1 -> Bus Creator5/1  "Outputs"
